simulink model "adaptive_fuzzy_control"  (R2024a)
settings: Solver=ode45  StartTime=0.0  StopTime=80  RelTol=1e-3
InitFcn:
  | Pp = [15 5; 5 5];
  | pnp = Pp(:, end);
  | Pa = [25 3; 3 3.8];
  | pna = Pa(:, end);
  | gamma_p = 2.5;
  | gamma_a = 100;
libraries: simulink x1
settings Model: Creator=dell 5550  LastModifiedBy=dell 5550

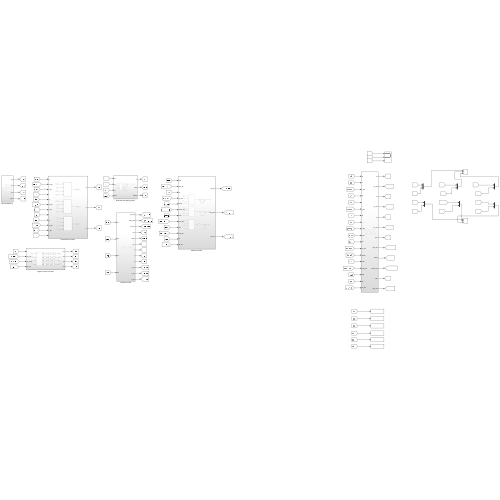
[thumbnail: Simulink's stored preview of the top-level diagram]
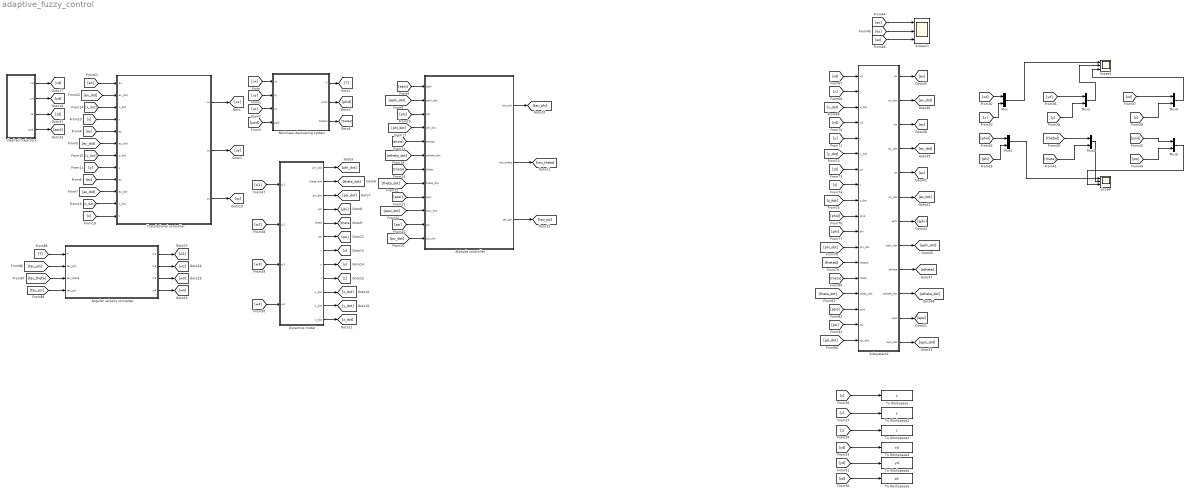
== system adaptive_fuzzy_control ==
  Angular velocity converter : Subsystem
  Attitude controller : Subsystem
  Desired trajectory : Subsystem
  Dynamics model : Subsystem
  Mux{,1..5} (6 alike) : Mux  Inputs=2
  Nonlinear decoupling system : Subsystem
  Scope : Scope  NumInputPorts=3
  Scope1 : Scope  NumInputPorts=3
  Scope11 : Scope  NumInputPorts=3
  Subsystem2 : Subsystem
  To Workspace : ToWorkspace  VariableName=x  SaveFormat=Timeseries  SampleTime=-1
  To Workspace1 : ToWorkspace  VariableName=y  SaveFormat=Timeseries  SampleTime=-1
  To Workspace2 : ToWorkspace  VariableName=z  SaveFormat=Timeseries  SampleTime=-1
  To Workspace3 : ToWorkspace  VariableName=xd  SaveFormat=Timeseries  SampleTime=-1
  To Workspace4 : ToWorkspace  VariableName=yd  SaveFormat=Timeseries  SampleTime=-1
  To Workspace5 : ToWorkspace  VariableName=zd  SaveFormat=Timeseries  SampleTime=-1
  Translational controller : Subsystem
  wires:
  Dynamics model/5(theta) -> [theta]
  Dynamics model/11(y_dot) -> [y_dot]
  Dynamics model/8(y) -> [y]
  Dynamics model/9(z) -> [z]
  Dynamics model/2(theta_dot) -> [theta_dot]
  Dynamics model/10(x_dot) -> [x_dot]
  Dynamics model/7(x) -> [x]
  Dynamics model/12(z_dot) -> [z_dot]
  Dynamics model/1(phi_dot) -> [phi_dot]
  Dynamics model/6(psi) -> [psi]
  Dynamics model/4(phi) -> [phi]
  Dynamics model/3(psi_dot) -> [psi_dot]
  Subsystem2/9(etheta) -> [etheta]
  Desired trajectory/3(zd) -> [zd]
  [x_dot] -> Subsystem2/3(x_dot)
  Desired trajectory/4(psid) -> [psid]
  [thetad] -> Subsystem2/13(thetad)
  Subsystem2/4(ey_dot) -> [ey_dot]
  [phid] -> Subsystem2/10(phid)
  Subsystem2/11(epsi) -> [epsi]
  Desired trajectory/2(yd) -> [yd]
  [psid] -> Subsystem2/16(psid)
  Subsystem2/10(etheta_dot) -> [etheta_dot]
  Subsystem2/12(epsi_dot) -> [epsi_dot]
  Subsystem2/1(ex) -> [ex]
  Subsystem2/2(ex_dot) -> [ex_dot]
  [z_dot] -> Subsystem2/9(z_dot)
  [zd] -> Subsystem2/7(zd)
  [y_dot] -> Subsystem2/6(y_dot)
  [x] -> Subsystem2/2(x)
  [z] -> Subsystem2/8(z)
  Subsystem2/7(ephi) -> [ephi]
  [xd] -> Subsystem2/1(xd)
  Subsystem2/3(ey) -> [ey]
  Desired trajectory/1(xd) -> [xd]
  [y] -> Subsystem2/5(y)
  Subsystem2/6(ez_dot) -> [ez_dot]
  Subsystem2/8(ephi_dot) -> [ephi_dot]
  [phi] -> Subsystem2/11(phi)
  [theta_dot] -> Subsystem2/15(theta_dot)
  Subsystem2/5(ez) -> [ez]
  [phi_dot] -> Subsystem2/12(phi_dot)
  [yd] -> Subsystem2/4(yd)
  [psi_dot] -> Subsystem2/18(psi_dot)
  [theta] -> Subsystem2/14(theta)
  [psi] -> Subsystem2/17(psi)
  [x] -> To Workspace/1
  [y] -> To Workspace1/1
  [z] -> To Workspace2/1
  [yd] -> To Workspace4/1
  [zd] -> To Workspace5/1
  [xd] -> To Workspace3/1
  [xd] -> Mux/1
  [x] -> Mux/2
  [phid] -> Mux1/1
  [phi] -> Mux1/2
  [yd] -> Mux3/1
  [y] -> Mux3/2
  [thetad] -> Mux2/1
  [theta] -> Mux2/2
  [zd] -> Mux4/1
  [z] -> Mux4/2
  [psid] -> Mux5/1
  [psi] -> Mux5/2
  Mux/1 -> Scope1/1
  Mux3/1 -> Scope1/2
  Mux4/1 -> Scope1/3
  Mux1/1 -> Scope/1
  Mux2/1 -> Scope/2
  Mux5/1 -> Scope/3
  [ex] -> Scope11/1
  [ey] -> Scope11/2
  [ez] -> Scope11/3
  [ex] -> Translational controller/1(ex)
  [ex_dot] -> Translational controller/2(ex_dot)
  [x] -> Translational controller/4(x)
  [x_dot] -> Translational controller/3(x_dot)
  [ey] -> Translational controller/5(ey)
  [ey_dot] -> Translational controller/6(ey_dot)
  [y_dot] -> Translational controller/7(y_dot)
  [y] -> Translational controller/8(y)
  [ez] -> Translational controller/9(ez)
  [ez_dot] -> Translational controller/10(ez_dot)
  [z_dot] -> Translational controller/11(z_dot)
  [z] -> Translational controller/12(z)
  Translational controller/1(ux) -> [ux]
  Translational controller/2(uy) -> [uy]
  Translational controller/3(uz) -> [uz]
  [ux] -> Nonlinear decoupling system/1(ux)
  [uy] -> Nonlinear decoupling system/2(uy)
  [uz] -> Nonlinear decoupling system/3(uz)
  [psid] -> Nonlinear decoupling system/4(psid)
  Nonlinear decoupling system/1(T) -> [T]
  Nonlinear decoupling system/2(phid) -> [phid]
  Nonlinear decoupling system/3(thetad) -> [thetad]
  [ephi] -> Attitude controller/1(ephi)
  [ephi_dot] -> Attitude controller/2(ephi_dot)
  [phi] -> Attitude controller/3(phi)
  [phi_dot] -> Attitude controller/4(phi_dot)
  [etheta] -> Attitude controller/5(etheta)
  [etheta_dot] -> Attitude controller/6(etheta_dot)
  [theta] -> Attitude controller/7(theta)
  [theta_dot] -> Attitude controller/8(theta_dot)
  [epsi] -> Attitude controller/9(epsi)
  [epsi_dot] -> Attitude controller/10(epsi_dot)
  [psi] -> Attitude controller/11(psi)
  [psi_dot] -> Attitude controller/12(psi_dot)
  Attitude controller/1(tau_phi) -> [tau_phi]
  Attitude controller/2(tau_theta) -> [tau_theta]
  Attitude controller/3(tau_psi) -> [tau_psi]
  [T] -> Angular velocity converter/1(T)
  [tau_phi] -> Angular velocity converter/2(tau_phi)
  [tau_theta] -> Angular velocity converter/3(tau_theta)
  [tau_psi] -> Angular velocity converter/4(tau_psi)
  Angular velocity converter/1(w1) -> [w1]
  Angular velocity converter/2(w2) -> [w2]
  Angular velocity converter/3(w3) -> [w3]
  Angular velocity converter/4(w4) -> [w4]
  [w1] -> Dynamics model/1(w1)
  [w2] -> Dynamics model/2(w2)
  [w3] -> Dynamics model/3(w3)
  [w4] -> Dynamics model/4(w4)

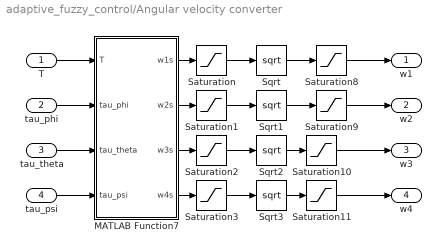
== system adaptive_fuzzy_control/Angular velocity converter ==
  T : Inport
  tau_phi : Inport  Port=2
  tau_theta : Inport  Port=3
  tau_psi : Inport  Port=4
  MATLAB Function7 : MATLAB Function  TreatAsAtomicUnit=on
  Saturation{,1..3} (4 alike) : Saturate  UpperLimit=inf  LowerLimit=0  ZeroCross=off
  Saturation{8..11} (4 alike) : Saturate  UpperLimit=1000  LowerLimit=0  ZeroCross=off
  Sqrt{,1..3} (4 alike) : Sqrt
  w1 : Outport
  w2 : Outport  Port=2
  w3 : Outport  Port=3
  w4 : Outport  Port=4
  wires:
  Saturation2/1 -> Sqrt2/1
  Sqrt3/1 -> Saturation11/1
  MATLAB Function7/1(w1s) -> Saturation/1
  Sqrt2/1 -> Saturation10/1
  Sqrt1/1 -> Saturation9/1
  Saturation1/1 -> Sqrt1/1
  tau_theta/1 -> MATLAB Function7/3(tau_theta)
  tau_psi/1 -> MATLAB Function7/4(tau_psi)
  Saturation/1 -> Sqrt/1
  Saturation3/1 -> Sqrt3/1
  MATLAB Function7/4(w4s) -> Saturation3/1
  Saturation10/1 -> w3/1
  MATLAB Function7/2(w2s) -> Saturation1/1
  Sqrt/1 -> Saturation8/1
  MATLAB Function7/3(w3s) -> Saturation2/1
  tau_phi/1 -> MATLAB Function7/2(tau_phi)
  T/1 -> MATLAB Function7/1(T)
  Saturation8/1 -> w1/1
  Saturation9/1 -> w2/1
  Saturation11/1 -> w4/1

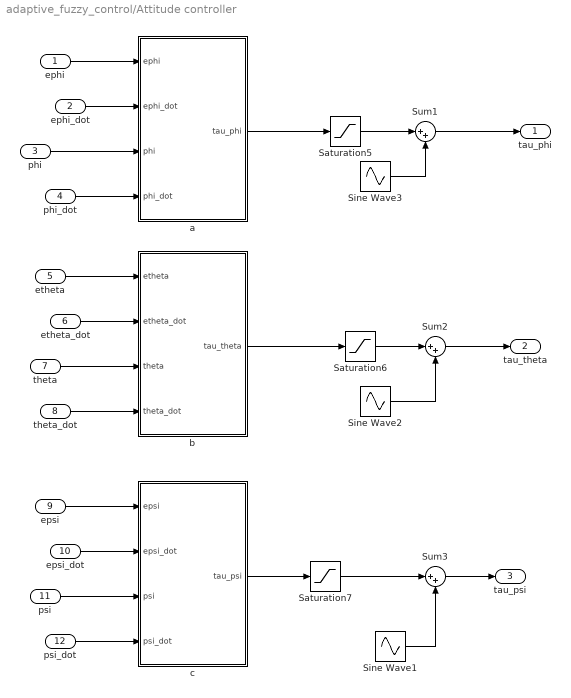
== system adaptive_fuzzy_control/Attitude controller ==
  ephi : Inport
  ephi_dot : Inport  Port=2
  phi : Inport  Port=3
  phi_dot : Inport  Port=4
  etheta : Inport  Port=5
  etheta_dot : Inport  Port=6
  theta : Inport  Port=7
  theta_dot : Inport  Port=8
  epsi : Inport  Port=9
  epsi_dot : Inport  Port=10
  psi : Inport  Port=11
  psi_dot : Inport  Port=12
  Saturation5 : Saturate  UpperLimit=3  LowerLimit=-3  ZeroCross=off
  Saturation6 : Saturate  UpperLimit=3  LowerLimit=-3  ZeroCross=off
  Saturation7 : Saturate  UpperLimit=0.05  LowerLimit=-0.05  ZeroCross=off
  Sine Wave1 : Sin  Amplitude=0.01  Phase=pi/2  SampleTime=0
  Sine Wave2 : Sin  Amplitude=0.03  Frequency=0.5  SampleTime=0
  Sine Wave3 : Sin  Amplitude=0.03  Frequency=0.5  Phase=pi/2  SampleTime=0
  Sum1 : Sum  Inputs=|++
  Sum2 : Sum  Inputs=|++
  Sum3 : Sum  Inputs=|++
  a : Subsystem
  b : Subsystem
  c : Subsystem
  tau_phi : Outport
  tau_theta : Outport  Port=2
  tau_psi : Outport  Port=3
  wires:
  b/1(tau_theta) -> Saturation6/1
  a/1(tau_phi) -> Saturation5/1
  c/1(tau_psi) -> Saturation7/1
  Saturation7/1 -> Sum3/1
  Saturation6/1 -> Sum2/1
  Sine Wave3/1 -> Sum1/2
  Saturation5/1 -> Sum1/1
  Sine Wave2/1 -> Sum2/2
  Sine Wave1/1 -> Sum3/2
  phi_dot/1 -> a/4(phi_dot)
  ephi/1 -> a/1(ephi)
  theta_dot/1 -> b/4(theta_dot)
  phi/1 -> a/3(phi)
  etheta_dot/1 -> b/2(etheta_dot)
  theta/1 -> b/3(theta)
  psi_dot/1 -> c/4(psi_dot)
  etheta/1 -> b/1(etheta)
  Sum1/1 -> tau_phi/1
  psi/1 -> c/3(psi)
  ephi_dot/1 -> a/2(ephi_dot)
  Sum2/1 -> tau_theta/1
  Sum3/1 -> tau_psi/1
  epsi/1 -> c/1(epsi)
  epsi_dot/1 -> c/2(epsi_dot)

== system adaptive_fuzzy_control/Desired trajectory ==
  Constant1 : Constant  Value=0
  Constant4 : Constant
  Ramp : simulink/Sources/Ramp  slope=0.025  start=0  InitialOutput=0
  Sine Wave : Sin  Amplitude=0.5  Frequency=pi/10  Phase=pi/2  SampleTime=0
  Sine Wave1 : Sin  Amplitude=0.5  Frequency=pi/10  SampleTime=0
  xd : Outport
  yd : Outport  Port=2
  zd : Outport  Port=3
  psid : Outport  Port=4
  wires:
  Constant1/1 -> psid/1
  Sine Wave/1 -> xd/1
  Sine Wave1/1 -> yd/1
  Ramp/1 -> zd/1

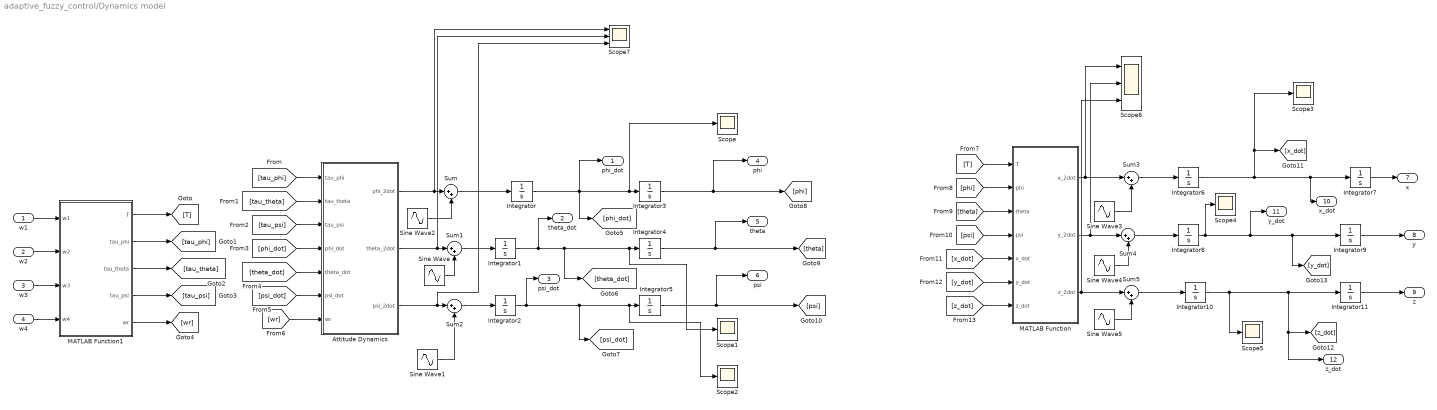
== system adaptive_fuzzy_control/Dynamics model ==
  w1 : Inport
  w2 : Inport  Port=2
  w3 : Inport  Port=3
  w4 : Inport  Port=4
  Attitude Dynamics : MATLAB Function  TreatAsAtomicUnit=on
  Integrator{,1..11} (12 alike) : Integrator
  MATLAB Function : MATLAB Function  TreatAsAtomicUnit=on
  MATLAB Function1 : MATLAB Function  TreatAsAtomicUnit=on
  Scope{,1..5} (6 alike) : Scope
  Scope6 : Scope  NumInputPorts=3
  Scope7 : Scope  NumInputPorts=3
  Sine Wave : Sin  Amplitude=2  Frequency=2  SampleTime=0
  Sine Wave1 : Sin  Amplitude=0.2  SampleTime=0
  Sine Wave2 : Sin  Amplitude=2  Frequency=2  SampleTime=0
  Sine Wave3 : Sin  Amplitude=0.1  SampleTime=0
  Sine Wave4 : Sin  Amplitude=0.1  SampleTime=0
  Sine Wave5 : Sin  Amplitude=0.05  Frequency=0.5  Phase=pi/2  SampleTime=0
  Sum{,1..5} (6 alike) : Sum  Inputs=|++
  phi_dot : Outport
  theta_dot : Outport  Port=2
  psi_dot : Outport  Port=3
  phi : Outport  Port=4
  theta : Outport  Port=5
  psi : Outport  Port=6
  x : Outport  Port=7
  y : Outport  Port=8
  z : Outport  Port=9
  x_dot : Outport  Port=10
  y_dot : Outport  Port=11
  z_dot : Outport  Port=12
  wires:
  w1/1 -> MATLAB Function1/1(w1)
  w2/1 -> MATLAB Function1/2(w2)
  w3/1 -> MATLAB Function1/3(w3)
  w4/1 -> MATLAB Function1/4(w4)
  MATLAB Function1/1(T) -> [T]
  MATLAB Function1/2(tau_phi) -> [tau_phi]
  MATLAB Function1/3(tau_theta) -> [tau_theta]
  MATLAB Function1/4(tau_psi) -> [tau_psi]
  MATLAB Function1/5(wr) -> [wr]
  [tau_phi] -> Attitude Dynamics/1(tau_phi)
  Integrator/1 -> phi_dot/1, Scope/1, Integrator3/1, [phi_dot]
  Integrator2/1 -> psi_dot/1, Scope2/1, Integrator5/1, [psi_dot]
  Integrator1/1 -> [theta_dot], Scope1/1, Integrator4/1, theta_dot/1
  [tau_theta] -> Attitude Dynamics/2(tau_theta)
  [tau_psi] -> Attitude Dynamics/3(tau_psi)
  [phi_dot] -> Attitude Dynamics/4(phi_dot)
  [theta_dot] -> Attitude Dynamics/5(theta_dot)
  [psi_dot] -> Attitude Dynamics/6(psi_dot)
  [wr] -> Attitude Dynamics/7(wr)
  Integrator3/1 -> phi/1, [phi]
  Integrator4/1 -> theta/1, [theta]
  Integrator5/1 -> psi/1, [psi]
  [T] -> MATLAB Function/1(T)
  [phi] -> MATLAB Function/2(phi)
  [theta] -> MATLAB Function/3(theta)
  [psi] -> MATLAB Function/4(psi)
  [x_dot] -> MATLAB Function/5(x_dot)
  [y_dot] -> MATLAB Function/6(y_dot)
  [z_dot] -> MATLAB Function/7(z_dot)
  Integrator9/1 -> y/1
  Integrator11/1 -> z/1
  Integrator8/1 -> Scope4/1, y_dot/1, [y_dot], Integrator9/1
  Integrator7/1 -> x/1
  Integrator10/1 -> Scope5/1, z_dot/1, [z_dot], Integrator11/1
  Integrator6/1 -> [x_dot], Scope3/1, x_dot/1, Integrator7/1
  Attitude Dynamics/1(phi_2dot) -> Scope7/1, Sum/1
  Sum/1 -> Integrator/1
  Attitude Dynamics/2(theta_2dot) -> Scope7/2, Sum1/1
  Sum1/1 -> Integrator1/1
  Attitude Dynamics/3(psi_2dot) -> Scope7/3, Sum2/1
  Sum2/1 -> Integrator2/1
  Sum3/1 -> Integrator6/1
  Sum4/1 -> Integrator8/1
  Sum5/1 -> Integrator10/1
  MATLAB Function/2(y_2dot) -> Sum4/1, Scope6/2
  MATLAB Function/3(z_2dot) -> Scope6/3, Sum5/1
  MATLAB Function/1(x_2dot) -> Sum3/1, Scope6/1
  Sine Wave3/1 -> Sum3/2
  Sine Wave4/1 -> Sum4/2
  Sine Wave5/1 -> Sum5/2
  Sine Wave2/1 -> Sum/2
  Sine Wave/1 -> Sum1/2
  Sine Wave1/1 -> Sum2/2

== system adaptive_fuzzy_control/Nonlinear decoupling system ==
  ux : Inport
  uy : Inport  Port=2
  uz : Inport  Port=3
  psid : Inport  Port=4
  MATLAB Function6 : MATLAB Function  TreatAsAtomicUnit=on
  Saturation4 : Saturate  UpperLimit=100  LowerLimit=0  ZeroCross=off
  Sine Wave : Sin  Amplitude=0.5  SampleTime=0
  Sum : Sum  Inputs=|++
  T : Outport
  phid : Outport  Port=2
  thetad : Outport  Port=3
  wires:
  ux/1 -> MATLAB Function6/1(ux)
  uz/1 -> MATLAB Function6/3(uz)
  Sum/1 -> T/1
  Saturation4/1 -> Sum/1
  MATLAB Function6/2(phid) -> phid/1
  MATLAB Function6/3(thetad) -> thetad/1
  MATLAB Function6/1(T) -> Saturation4/1
  Sine Wave/1 -> Sum/2
  psid/1 -> MATLAB Function6/4(psid)
  uy/1 -> MATLAB Function6/2(uy)

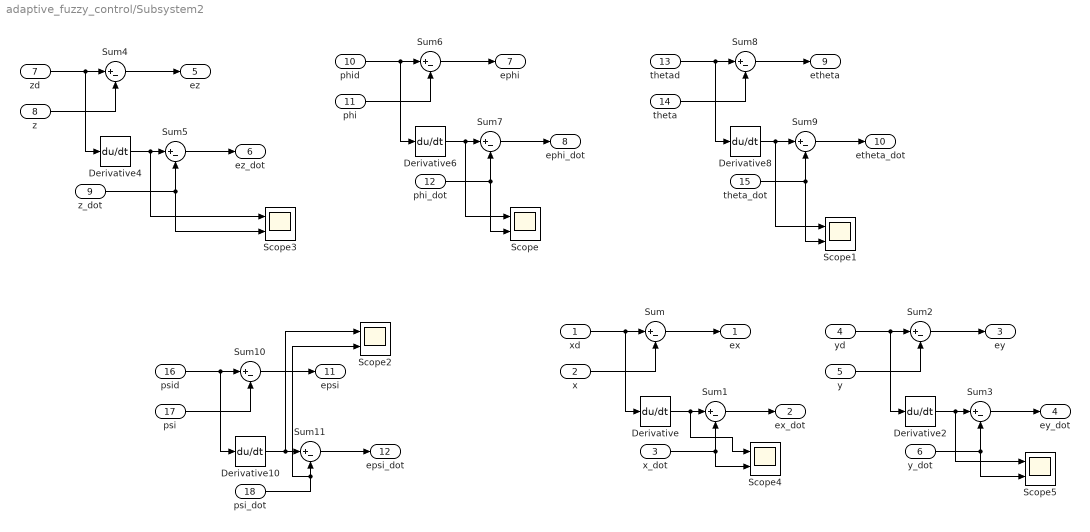
== system adaptive_fuzzy_control/Subsystem2 ==
  xd : Inport
  x : Inport  Port=2
  x_dot : Inport  Port=3
  yd : Inport  Port=4
  y : Inport  Port=5
  y_dot : Inport  Port=6
  zd : Inport  Port=7
  z : Inport  Port=8
  z_dot : Inport  Port=9
  phid : Inport  Port=10
  phi : Inport  Port=11
  phi_dot : Inport  Port=12
  thetad : Inport  Port=13
  theta : Inport  Port=14
  theta_dot : Inport  Port=15
  psid : Inport  Port=16
  psi : Inport  Port=17
  psi_dot : Inport  Port=18
  Derivative{,2,4,6,8,10} (6 alike) : Derivative  CoefficientInTFapproximation=0.001
  Scope{,1..5} (6 alike) : Scope  NumInputPorts=2
  Sum{,1..11} (12 alike) : Sum  Inputs=|+-
  ex : Outport
  ex_dot : Outport  Port=2
  ey : Outport  Port=3
  ey_dot : Outport  Port=4
  ez : Outport  Port=5
  ez_dot : Outport  Port=6
  ephi : Outport  Port=7
  ephi_dot : Outport  Port=8
  etheta : Outport  Port=9
  etheta_dot : Outport  Port=10
  epsi : Outport  Port=11
  epsi_dot : Outport  Port=12
  wires:
  xd/1 -> Derivative/1, Sum/1
  x/1 -> Sum/2
  Sum/1 -> ex/1
  Derivative/1 -> Scope4/1, Sum1/1
  x_dot/1 -> Scope4/2, Sum1/2
  Sum1/1 -> ex_dot/1
  Sum3/1 -> ey_dot/1
  y_dot/1 -> Scope5/2, Sum3/2
  Derivative2/1 -> Scope5/1, Sum3/1
  Sum2/1 -> ey/1
  y/1 -> Sum2/2
  yd/1 -> Sum2/1, Derivative2/1
  zd/1 -> Derivative4/1, Sum4/1
  z/1 -> Sum4/2
  Sum4/1 -> ez/1
  Derivative4/1 -> Scope3/1, Sum5/1
  z_dot/1 -> Scope3/2, Sum5/2
  Sum5/1 -> ez_dot/1
  Sum7/1 -> ephi_dot/1
  phi_dot/1 -> Scope/2, Sum7/2
  Derivative6/1 -> Scope/1, Sum7/1
  Sum6/1 -> ephi/1
  phi/1 -> Sum6/2
  phid/1 -> Sum6/1, Derivative6/1
  thetad/1 -> Derivative8/1, Sum8/1
  theta/1 -> Sum8/2
  Sum8/1 -> etheta/1
  Derivative8/1 -> Scope1/1, Sum9/1
  theta_dot/1 -> Scope1/2, Sum9/2
  Sum9/1 -> etheta_dot/1
  Sum11/1 -> epsi_dot/1
  psi_dot/1 -> Scope2/2, Sum11/2
  Derivative10/1 -> Scope2/1, Sum11/1
  Sum10/1 -> epsi/1
  psi/1 -> Sum10/2
  psid/1 -> Sum10/1, Derivative10/1

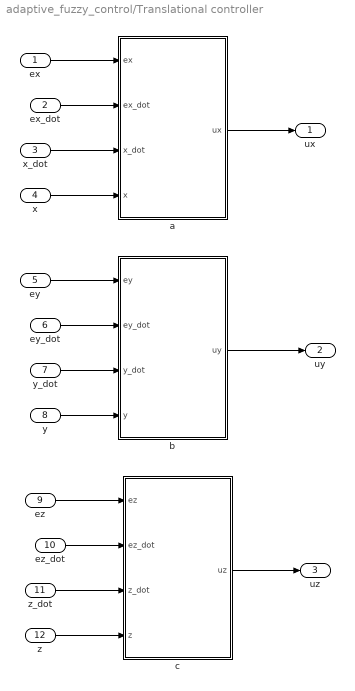
== system adaptive_fuzzy_control/Translational controller ==
  ex : Inport
  ex_dot : Inport  Port=2
  x_dot : Inport  Port=3
  x : Inport  Port=4
  ey : Inport  Port=5
  ey_dot : Inport  Port=6
  y_dot : Inport  Port=7
  y : Inport  Port=8
  ez : Inport  Port=9
  ez_dot : Inport  Port=10
  z_dot : Inport  Port=11
  z : Inport  Port=12
  a : Subsystem
  b : Subsystem
  c : Subsystem
  ux : Outport
  uy : Outport  Port=2
  uz : Outport  Port=3
  wires:
  x_dot/1 -> a/3(x_dot)
  b/1(uy) -> uy/1
  ez_dot/1 -> c/2(ez_dot)
  ey/1 -> b/1(ey)
  y_dot/1 -> b/3(y_dot)
  ex_dot/1 -> a/2(ex_dot)
  ez/1 -> c/1(ez)
  ex/1 -> a/1(ex)
  z/1 -> c/4(z)
  y/1 -> b/4(y)
  z_dot/1 -> c/3(z_dot)
  x/1 -> a/4(x)
  ey_dot/1 -> b/2(ey_dot)
  a/1(ux) -> ux/1
  c/1(uz) -> uz/1

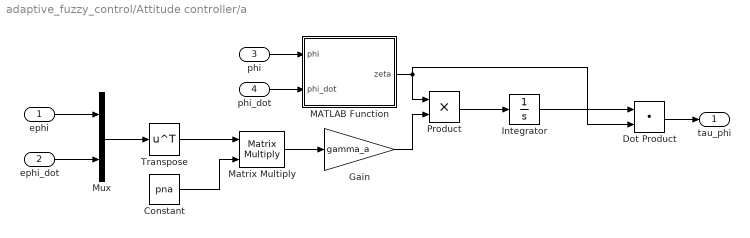
== system adaptive_fuzzy_control/Attitude controller/a ==
  ephi : Inport
  ephi_dot : Inport  Port=2
  phi : Inport  Port=3
  phi_dot : Inport  Port=4
  Constant : Constant  Value=pna
  Dot Product : DotProduct  OutDataTypeStr=Inherit: Inherit via internal rule
  Gain : Gain  Gain=gamma_a
  Integrator : Integrator
  MATLAB Function : MATLAB Function  TreatAsAtomicUnit=on
  Matrix Multiply : Product  Multiplication=Matrix(*)
  Mux : Mux  Inputs=2
  Product : Product
  Transpose : Math  Operator=transpose
  tau_phi : Outport
  wires:
  Dot Product/1 -> tau_phi/1
  Integrator/1 -> Dot Product/1
  MATLAB Function/1(zeta) -> Product/1, Dot Product/2
  Product/1 -> Integrator/1
  Gain/1 -> Product/2
  Matrix Multiply/1 -> Gain/1
  Transpose/1 -> Matrix Multiply/1
  Mux/1 -> Transpose/1
  Constant/1 -> Matrix Multiply/2
  ephi_dot/1 -> Mux/2
  ephi/1 -> Mux/1
  phi_dot/1 -> MATLAB Function/2(phi_dot)
  phi/1 -> MATLAB Function/1(phi)

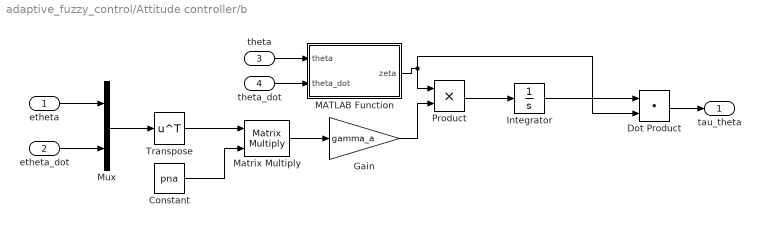
== system adaptive_fuzzy_control/Attitude controller/b ==
  etheta : Inport
  etheta_dot : Inport  Port=2
  theta : Inport  Port=3
  theta_dot : Inport  Port=4
  Constant : Constant  Value=pna
  Dot Product : DotProduct  OutDataTypeStr=Inherit: Inherit via internal rule
  Gain : Gain  Gain=gamma_a
  Integrator : Integrator
  MATLAB Function : MATLAB Function  TreatAsAtomicUnit=on
  Matrix Multiply : Product  Multiplication=Matrix(*)
  Mux : Mux  Inputs=2
  Product : Product
  Transpose : Math  Operator=transpose
  tau_theta : Outport
  wires:
  etheta/1 -> Mux/1
  etheta_dot/1 -> Mux/2
  Constant/1 -> Matrix Multiply/2
  Mux/1 -> Transpose/1
  Transpose/1 -> Matrix Multiply/1
  Matrix Multiply/1 -> Gain/1
  Gain/1 -> Product/2
  Product/1 -> Integrator/1
  theta_dot/1 -> MATLAB Function/2(theta_dot)
  MATLAB Function/1(zeta) -> Product/1, Dot Product/2
  Integrator/1 -> Dot Product/1
  Dot Product/1 -> tau_theta/1
  theta/1 -> MATLAB Function/1(theta)

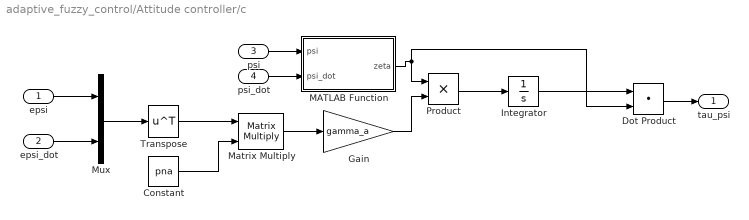
== system adaptive_fuzzy_control/Attitude controller/c ==
  epsi : Inport
  epsi_dot : Inport  Port=2
  psi : Inport  Port=3
  psi_dot : Inport  Port=4
  Constant : Constant  Value=pna
  Dot Product : DotProduct  OutDataTypeStr=Inherit: Inherit via internal rule
  Gain : Gain  Gain=gamma_a
  Integrator : Integrator
  MATLAB Function : MATLAB Function  TreatAsAtomicUnit=on
  Matrix Multiply : Product  Multiplication=Matrix(*)
  Mux : Mux  Inputs=2
  Product : Product
  Transpose : Math  Operator=transpose
  tau_psi : Outport
  wires:
  Dot Product/1 -> tau_psi/1
  Integrator/1 -> Dot Product/1
  MATLAB Function/1(zeta) -> Dot Product/2, Product/1
  Product/1 -> Integrator/1
  Gain/1 -> Product/2
  Matrix Multiply/1 -> Gain/1
  Transpose/1 -> Matrix Multiply/1
  Mux/1 -> Transpose/1
  Constant/1 -> Matrix Multiply/2
  epsi_dot/1 -> Mux/2
  epsi/1 -> Mux/1
  psi_dot/1 -> MATLAB Function/2(psi_dot)
  psi/1 -> MATLAB Function/1(psi)

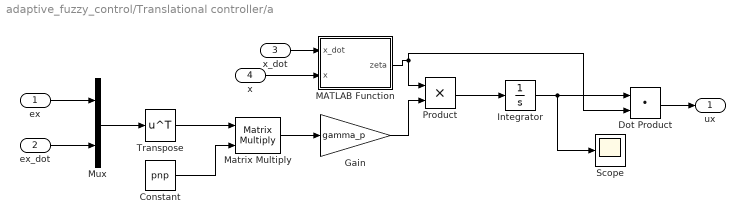
== system adaptive_fuzzy_control/Translational controller/a ==
  ex : Inport
  ex_dot : Inport  Port=2
  x_dot : Inport  Port=3
  x : Inport  Port=4
  Constant : Constant  Value=pnp
  Dot Product : DotProduct  OutDataTypeStr=Inherit: Inherit via internal rule
  Gain : Gain  Gain=gamma_p
  Integrator : Integrator
  MATLAB Function : MATLAB Function  TreatAsAtomicUnit=on
  Matrix Multiply : Product  Multiplication=Matrix(*)
  Mux : Mux  Inputs=2
  Product : Product
  Scope : Scope
  Transpose : Math  Operator=transpose
  ux : Outport
  wires:
  ex/1 -> Mux/1
  ex_dot/1 -> Mux/2
  Constant/1 -> Matrix Multiply/2
  Mux/1 -> Transpose/1
  Transpose/1 -> Matrix Multiply/1
  Matrix Multiply/1 -> Gain/1
  Gain/1 -> Product/2
  Product/1 -> Integrator/1
  x_dot/1 -> MATLAB Function/1(x_dot)
  MATLAB Function/1(zeta) -> Product/1, Dot Product/2
  Integrator/1 -> Dot Product/1, Scope/1
  Dot Product/1 -> ux/1
  x/1 -> MATLAB Function/2(x)

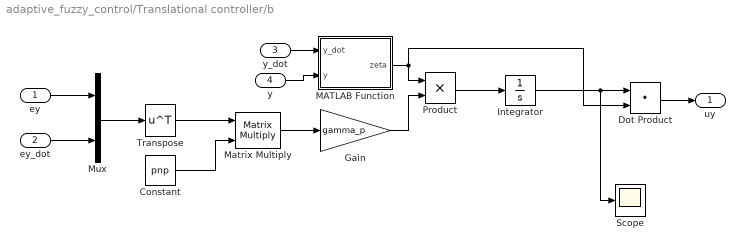
== system adaptive_fuzzy_control/Translational controller/b ==
  ey : Inport
  ey_dot : Inport  Port=2
  y_dot : Inport  Port=3
  y : Inport  Port=4
  Constant : Constant  Value=pnp
  Dot Product : DotProduct  OutDataTypeStr=Inherit: Inherit via internal rule
  Gain : Gain  Gain=gamma_p
  Integrator : Integrator
  MATLAB Function : MATLAB Function  TreatAsAtomicUnit=on
  Matrix Multiply : Product  Multiplication=Matrix(*)
  Mux : Mux  Inputs=2
  Product : Product
  Scope : Scope
  Transpose : Math  Operator=transpose
  uy : Outport
  wires:
  Dot Product/1 -> uy/1
  Integrator/1 -> Scope/1, Dot Product/1
  MATLAB Function/1(zeta) -> Dot Product/2, Product/1
  y_dot/1 -> MATLAB Function/1(y_dot)
  Product/1 -> Integrator/1
  Gain/1 -> Product/2
  Matrix Multiply/1 -> Gain/1
  Transpose/1 -> Matrix Multiply/1
  Mux/1 -> Transpose/1
  Constant/1 -> Matrix Multiply/2
  ey_dot/1 -> Mux/2
  ey/1 -> Mux/1
  y/1 -> MATLAB Function/2(y)

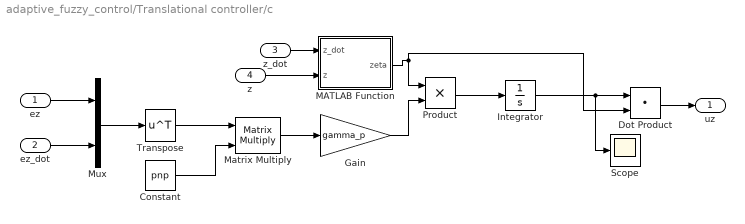
== system adaptive_fuzzy_control/Translational controller/c ==
  ez : Inport
  ez_dot : Inport  Port=2
  z_dot : Inport  Port=3
  z : Inport  Port=4
  Constant : Constant  Value=pnp
  Dot Product : DotProduct  OutDataTypeStr=Inherit: Inherit via internal rule
  Gain : Gain  Gain=gamma_p
  Integrator : Integrator
  MATLAB Function : MATLAB Function  TreatAsAtomicUnit=on
  Matrix Multiply : Product  Multiplication=Matrix(*)
  Mux : Mux  Inputs=2
  Product : Product
  Scope : Scope
  Transpose : Math  Operator=transpose
  uz : Outport
  wires:
  ez/1 -> Mux/1
  ez_dot/1 -> Mux/2
  Constant/1 -> Matrix Multiply/2
  Mux/1 -> Transpose/1
  Transpose/1 -> Matrix Multiply/1
  Matrix Multiply/1 -> Gain/1
  Gain/1 -> Product/2
  Product/1 -> Integrator/1
  z_dot/1 -> MATLAB Function/1(z_dot)
  MATLAB Function/1(zeta) -> Product/1, Dot Product/2
  Integrator/1 -> Scope/1, Dot Product/1
  Dot Product/1 -> uz/1
  z/1 -> MATLAB Function/2(z)

== matlab function adaptive_fuzzy_control/Translational controller/a/MATLAB Function ==
  data: x_dot input; zeta output; x input
function zeta  = fcn(x_dot, x)
    c_x_dot = -2:0.8:2;
    w_x_dot = 0.4;
    c_x = -2.5:1:2.5;
    w_x = 0.5;
    mu_x_dot = zeros(1, 6);
    for i = 1:6
        mu_x_dot(i) = exp(-(x_dot - c_x_dot(i))^2 / (2 * w_x_dot^2));
    end
    mu_x = zeros(1, 6);
    for i = 1:6
        mu_x(i) = exp(-(x - c_x(i))^2 / (2 * w_x^2));
    end
    zeta = zeros(36, 1);
    k = 1;
    for i = 1:6
        for j = 1:6
            zeta(k) = mu_x(i) * mu_x_dot(j);
            k = k + 1;
        end
    end
end

== matlab function adaptive_fuzzy_control/Nonlinear decoupling system/MATLAB Function6 ==
  data: ux input; uy input; T output; uz input; phid output; thetad output; psid input
function [T, phid, thetad] = fcn(ux, uy, uz, psid)
m = 1.121;
g = 9.81;
T = m*sqrt(ux^2 + uy^2 + (uz + g)^2);
phid = asin((ux * sin(psid) - uy * cos(psid)) / sqrt(ux^2 + uy^2 + (uz + g)^2));
thetad = atan((ux * cos(psid) + uy * sin(psid)) / (uz + g));

== matlab function adaptive_fuzzy_control/Angular velocity converter/MATLAB Function7 ==
  data: T input; w1s output; tau_phi input; tau_theta input; tau_psi input; w2s output; w3s output; w4s output
function [w1s, w2s, w3s, w4s] = fcn(T, tau_phi, tau_theta, tau_psi)
k = 2.98e-5;
b = 3.23e-7;
l = 0.25;
w1s = T/4/k - tau_theta/2/k/l - tau_psi/4/b;
w2s = T/4/k - tau_phi/2/k/l + tau_psi/4/b;
w3s = T/4/k + tau_theta/2/k/l - tau_psi/4/b;
w4s = T/4/k + tau_phi/2/k/l + tau_psi/4/b;

== matlab function adaptive_fuzzy_control/Translational controller/b/MATLAB Function ==
  data: y_dot input; zeta output; y input
function zeta  = fcn(y_dot, y)
    c_y_dot = -2:0.8:2;
    w_y_dot = 0.4;
    c_y = -2.5:1:2.5;
    w_y = 0.5;
    mu_y_dot = zeros(1, 6);
    for i = 1:6
        mu_y_dot(i) = exp(-(y_dot - c_y_dot(i))^2 / (2 * w_y_dot^2));
    end
    mu_y = zeros(1, 6);
    for i = 1:6
        mu_y(i) = exp(-(y - c_y(i))^2 / (2 * w_y^2));
    end
    zeta = zeros(36, 1);
    k = 1;
    for i = 1:6
        for j = 1:6
            zeta(k) = mu_y(i) * mu_y_dot(j);
            k = k + 1;
        end
    end
end

== matlab function adaptive_fuzzy_control/Dynamics model/Attitude Dynamics ==
  data: tau_phi input; phi_2dot output; tau_theta input; tau_psi input; phi_dot input; theta_dot input; psi_dot input; theta_2dot output; psi_2dot output; wr input
function [phi_2dot, theta_2dot, psi_2dot] = fcn(tau_phi, tau_theta, tau_psi, phi_dot, theta_dot, psi_dot, wr)
Ix = 0.01;
Iy = 0.01;
Iz = 0.0148;
Ir = 2.83e-5;
phi_2dot = (tau_phi + (Iy - Iz) * theta_dot * psi_dot - theta_dot * Ir * wr) / Ix;
theta_2dot = (tau_theta + (Iz - Ix) * phi_dot * psi_dot + phi_dot * Ir * wr) / Iy;
psi_2dot = (tau_psi + (Ix - Iy) * theta_dot * phi_dot ) / Iz;

== matlab function adaptive_fuzzy_control/Dynamics model/MATLAB Function1 ==
  data: w1 input; T output; w2 input; w3 input; w4 input; tau_phi output; tau_theta output; tau_psi output; wr output
function [T, tau_phi, tau_theta, tau_psi, wr] = fcn(w1, w2, w3, w4)
k = 2.98e-5;
b = 3.23e-7;
l = 0.25;
T = k * (w1^2 + w2^2 + w3^2 + w4^2);
tau_phi = k * l * (w4^2 - w2^2);
tau_theta = k * l * (w3^2 - w1^2);
tau_psi = b * (w4^2 + w2^2 - w3^2 - w1^2);
wr = w1 - w2 + w3 - w4;

== matlab function adaptive_fuzzy_control/Dynamics model/MATLAB Function ==
  data: T input; x_2dot output; phi input; theta input; psi input; x_dot input; y_dot input; z_dot input; y_2dot output; z_2dot output
function [x_2dot, y_2dot, z_2dot] = fcn(T, phi, theta, psi, x_dot, y_dot, z_dot)
Ax = 5.56e-4;
Ay = 5.56e-4;
Az = 6.35e-4;
m = 1.121;
g = 9.81;
x_2dot = T / m * (cos(phi) * sin(theta) * cos(psi) + sin(phi) * sin(psi)) - Ax * x_dot / m;
y_2dot = T / m * (cos(phi) * sin(theta) * sin(psi) - sin(phi) * cos(psi)) - Ay * y_dot / m;
z_2dot = T / m * cos(phi) * cos(theta) - g - Az * z_dot / m;

== matlab function adaptive_fuzzy_control/Translational controller/c/MATLAB Function ==
  data: z_dot input; zeta output; z input
function zeta  = fcn(z_dot, z)
    c_z_dot = -1.5:0.6:1.5;
    w_z_dot = 0.3;
    c_z = 0:0.6:3;
    w_z = 0.3;
    mu_z_dot = zeros(1, 6);
    for i = 1:6
        mu_z_dot(i) = exp(-(z_dot - c_z_dot(i))^2 / (2 * w_z_dot^2));
    end
    mu_z = zeros(1, 6);
    for i = 1:6
        mu_z(i) = exp(-(z - c_z(i))^2 / (2 * w_z^2));
    end
    zeta = zeros(36, 1);
    k = 1;
    for i = 1:6
        for j = 1:6
            zeta(k) = mu_z(i) * mu_z_dot(j);
            k = k + 1;
        end
    end
end

== matlab function adaptive_fuzzy_control/Attitude controller/a/MATLAB Function ==
  data: phi input; zeta output; phi_dot input
function zeta  = fcn(phi, phi_dot)
    c_phi = -pi/9:pi/18:pi/9;
    w_phi = pi/36;
    c_phi_dot = -1.5:0.6:1.5;
    w_phi_dot = 0.3;

    mu_phi = zeros(1, 5);
    for i = 1:5
        mu_phi(i) = exp(-(phi - c_phi(i))^2 / (2 * w_phi^2));
    end

    mu_phi_dot = zeros(1, 6);
    for i = 1:6
        mu_phi_dot(i) = exp(-(phi_dot - c_phi_dot(i))^2 / (2 * w_phi_dot^2));
    end

    zeta = zeros(30, 1);
    k = 1;
    for i = 1:5
        for j = 1:6
            zeta(k) = mu_phi(i) * mu_phi_dot(j);
            k = k + 1;
        end
    end
end

== matlab function adaptive_fuzzy_control/Attitude controller/b/MATLAB Function ==
  data: theta input; theta_dot input; zeta output
function zeta  = fcn(theta, theta_dot)
    c_theta = -pi/9:pi/18:pi/9;
    w_theta = pi/36;
    c_theta_dot = -1.5:0.6:1.5;
    w_theta_dot = 0.3;
    mu_theta_dot = zeros(1, 6);
    for i = 1:5
        mu_theta_dot(i) = exp(-(theta_dot - c_theta_dot(i))^2 / (2 * w_theta_dot^2));
    end

    mu_theta = zeros(1, 5);
    for i = 1:5
        mu_theta(i) = exp(-(theta - c_theta(i))^2 / (2 * w_theta^2));
    end

    zeta = zeros(30, 1);
    k = 1;
    for i = 1:5
        for j = 1:6
            zeta(k) = mu_theta(i) * mu_theta_dot(j);
            k = k + 1;
        end
    end
end

== matlab function adaptive_fuzzy_control/Attitude controller/c/MATLAB Function ==
  data: psi input; psi_dot input; zeta output
function zeta  = fcn(psi, psi_dot)
    c_psi = -0.001:0.0005:0.001;
    w_psi = 0.00025;
    c_psi_dot = -0.01:0.004:0.01;
    w_psi_dot = 0.002;
    mu_psi_dot = zeros(1, 6);
    for i = 1:6
        mu_psi_dot(i) = exp(-(psi_dot - c_psi_dot(i))^2 / (2 * w_psi_dot^2));
    end

    mu_psi = zeros(1, 5);
    for i = 1:5
        mu_psi(i) = exp(-(psi - c_psi(i))^2 / (2 * w_psi^2));
    end

    zeta = zeros(30, 1);
    k = 1;
    for i = 1:5
        for j = 1:6
            zeta(k) = mu_psi(i) * mu_psi_dot(j);
            k = k + 1;
        end
    end
end
